simulink model "gps_direct"  (R2024b)
settings: Solver=FixedStepAuto  StartTime=0.0  StopTime=inf  FixedStep=0.05  RelTol=1e-3
libraries: arduinolib x1
settings Model: ExtModeTrigDuration=2  Creator=Nitesh  LastModifiedBy=Nitesh
settings SolverCC: AutoInsertRateTranBlk=on
settings OptimizationCC: EnhancedBackFolding=on  PassReuseOutputArgsAs=Individual arguments  ZeroExternalMemoryAtStartup=off  ZeroInternalMemoryAtStartup=off  MaxStackSize=64  OptimizeBlockOrder=speed  DifferentSizesBufferReuse=on  OptimizationCustomize=off  EfficientTunableParamExpr=on
settings DebuggingCC: ParameterTunabilityLossMsg=error
settings HardwareCC: ProdBitPerPointer=32  ProdBitPerSizeT=32  ProdBitPerPtrDiffT=32  ProdLargestAtomicInteger=Long  ProdLargestAtomicFloat=Double  ProdWordSize=32  ProdHWDeviceType=ARM Compatible->ARM Cortex  UseEmbeddedCoderFeatures=off
settings RTWCC: Description=Embedded Coder  SystemTargetFile=ert.tlc  HardwareBoard=ESP32-WROOM(Arduino Compatible)  TLCOptions="-aInlineSetEventsForThisBaseRateFcn=TLC_FALSE -aSuppressMultiTaskScheduler=TLC_FALSE  -aRateBasedStepFcn=0"  TemplateMakefile=ert_default_tmf  Toolchain=ESP32
settings CodeAppCC: ForceParamTrailComments=on  IgnoreCustomStorageClasses=off  OperatorAnnotations=on  SimulinkDataObjDesc=on  SFDataObjDesc=on  InsertBlockDesc=on
settings ERTTargetCC: SupportContinuousTime=on  SupportNonInlinedSFcns=on  SupportVariableSizeSignals=on  ExtModeTransport=3  ExtModeStaticAlloc=on  ExtModeAutomaticAllocSize=off  ExtModeStaticAllocSize=65536  ExtModeMexFile=ext_xcp  ExtModeIntrfLevel=Level2 - Open  InlinedParameterPlacement=Hierarchical

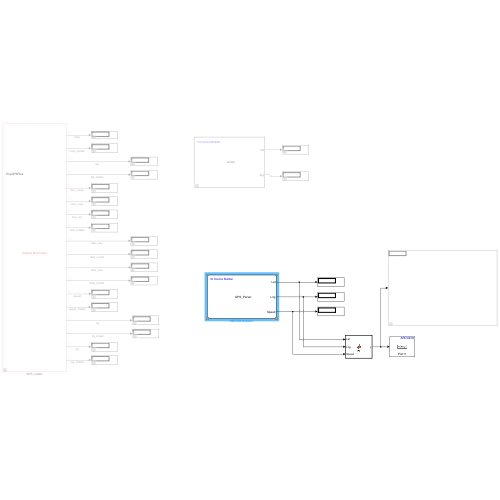
[thumbnail: Simulink's stored preview of the top-level diagram]
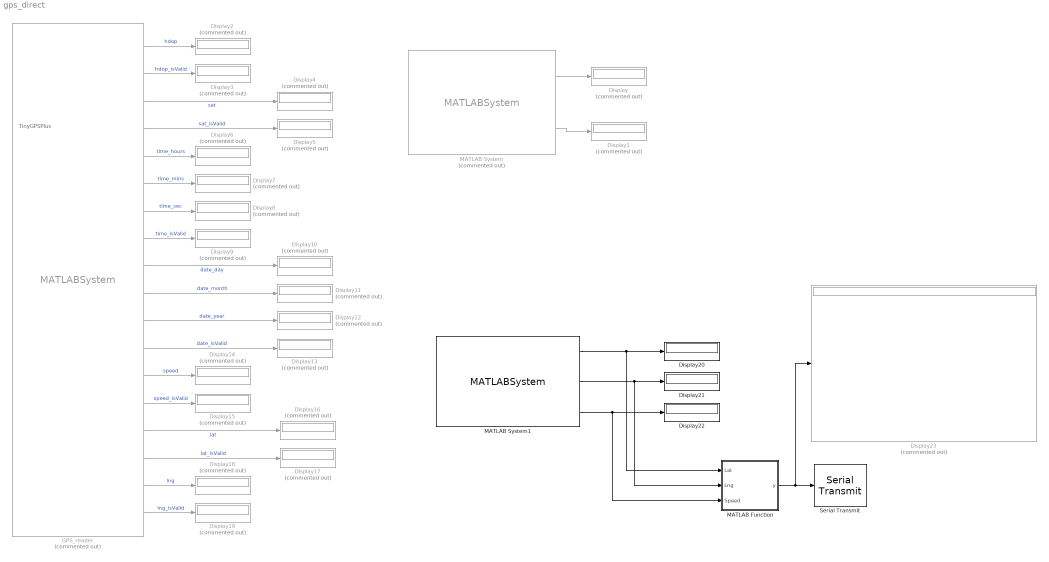
== system gps_direct ==
  note: TinyGPSPlus
  Display{,1..19,23} (21 alike) : Display  Commented=on
  Display20 : Display
  Display21 : Display
  Display22 : Display
  GPS_reader : MATLABSystem  Commented=on  System=gps_reader  SampleTime=500e-3
  MATLAB Function : MATLAB Function  TreatAsAtomicUnit=on
  MATLAB System : MATLABSystem  Commented=on  System=reader  SampleTime=1
      mask Type: reader
      mask Display:
      | color('white');plot([100,100,100,100]*1,[100,100,100,100]*1);plot([100,100,100,100]*0,[100,100,100,100]*0);color('blue');text(38, 92, 'IO Device Builder','horizontalAlignment', 'right');
      | color('black');text(52,50,' reader','horizontalAlignment','center');
      | port_label('output',1,'lat');port_label('output',2,'lng');
  MATLAB System1 : MATLABSystem  System=GPS_Parser  SampleTime=0.050
      mask Type: GPS_Parser
      mask Display:
      | color('white');plot([100,100,100,100]*1,[100,100,100,100]*1);plot([100,100,100,100]*0,[100,100,100,100]*0);color('blue');text(38, 92, 'IO Device Builder','horizontalAlignment', 'right');
      | color('black');text(52,50,' GPS_Parser','horizontalAlignment','center');
      | port_label('output',1,'Lat');port_label('output',2,'Lng');port_label('output',3,'Speed');
  Serial Transmit : arduinolib/Serial Transmit  portNumber=0  sendmode=write  sendformat=Decimal  floatprecision=2  header=[]  terminator=[]  blockPlatform=ARDUINO
      settings: SourceProductName=Common
  wires:
  MATLAB System/1 -> Display/1
  MATLAB System/2 -> Display1/1
  GPS_reader/1 -> Display2/1  "hdop"
  GPS_reader/2 -> Display3/1  "hdop_isValid"
  GPS_reader/4 -> Display5/1  "sat_isValid"
  GPS_reader/3 -> Display4/1  "sat"
  GPS_reader/6 -> Display7/1  "time_mins"
  GPS_reader/5 -> Display6/1  "time_hours"
  GPS_reader/7 -> Display8/1  "time_sec"
  GPS_reader/8 -> Display9/1  "time_isValid"
  GPS_reader/12 -> Display13/1  "date_isValid"
  GPS_reader/11 -> Display12/1  "date_year"
  GPS_reader/9 -> Display10/1  "date_day"
  GPS_reader/10 -> Display11/1  "date_month"
  GPS_reader/14 -> Display15/1  "speed_isValid"
  GPS_reader/13 -> Display14/1  "speed"
  GPS_reader/15 -> Display16/1  "lat"
  GPS_reader/16 -> Display17/1  "lat_isValid"
  GPS_reader/17 -> Display18/1  "lng"
  GPS_reader/18 -> Display19/1  "lng_isValid"
  MATLAB System1/1 -> MATLAB Function/1(Lat), Display20/1
  MATLAB System1/2 -> MATLAB Function/2(Lng), Display21/1
  MATLAB System1/3 -> Display22/1, MATLAB Function/3(Speed)
  MATLAB Function/1(y) -> Display23/1, Serial Transmit/1

== matlab function gps_direct/MATLAB Function ==
  data: Lat input; y output uint8 size=[1 60]; Lng input; Speed input double
function y = fcn(Lat, Lng, Speed)
    str = blanks(60);

    message = sprintf('\nLat: %.7f, Lng: %.7f Speed: %.7f', Lat, Lng, Speed);

    str(1:length(message)) = message;
    y = uint8(str);
